simulink model "Simplified_Model_test"  (R2014a)
settings: Solver=ode45  StartTime=0.0  StopTime=10.0  RelTol=1e-3
libraries: simulink x3, rocket_vertical_flight_library x1
settings Model: Creator=scorpii  LastModifiedBy=scorpii

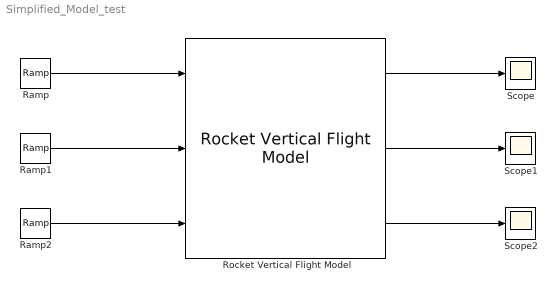
== system Simplified_Model_test ==
  Ramp : simulink/Sources/Ramp  slope=2  start=0  X0=0
  Ramp1 : simulink/Sources/Ramp  slope=-1  start=0  X0=5
  Ramp2 : simulink/Sources/Ramp  slope=0.5  start=0  X0=0
  Rocket Vertical Flight Model : rocket_vertical_flight_library/Rocket Vertical Flight Model
  Scope : Scope
  Scope1 : Scope
  Scope2 : Scope
      settings: SaveName=ScopeData2
  wires:
  Ramp/1 -> Rocket Vertical Flight Model/1
  Rocket Vertical Flight Model/1 -> Scope/1
  Rocket Vertical Flight Model/2 -> Scope1/1
  Rocket Vertical Flight Model/3 -> Scope2/1
  Ramp1/1 -> Rocket Vertical Flight Model/2
  Ramp2/1 -> Rocket Vertical Flight Model/3
